simulink model "GalvoModel_v3_tfCCneu"  (R2013a)
settings: Solver=ode45  StartTime=0.0  StopTime=1.5  RelTol=1e-3
undefined symbols (not defined in the file or in its folder): BEM, ccKp, CL, CR, FR, H, KTR, RIN, TRC
libraries: simulink x1
settings Model: Creator=mainster  LastModifiedBy=mainster
settings DebuggingCC: SolverPrmCheckMsg=none

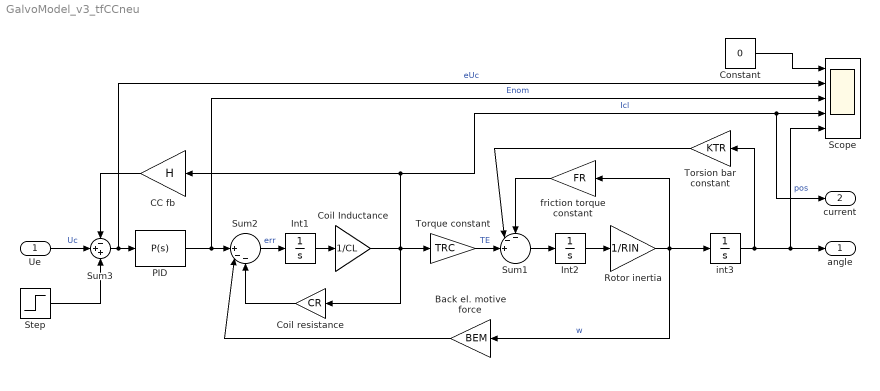
== system GalvoModel_v3_tfCCneu ==
  Ue : Inport
  Back el. motive force : Gain  Gain=BEM
  CC fb : Gain  StartFcn=|  Gain=H
      | %H=100;                       
      | sprintf('StartFcn: H is %i',H)
      settings: AttributesFormatString=H=eval(%<Gain>)
  Coil Inductance : Gain  Gain=1/CL
  Coil resistance : Gain  Gain=CR
  Constant : Constant  Value=0
  Int1 : Integrator
  Int2 : Integrator
  PID : simulink/Continuous/PID Controller  Controller=P  TimeDomain=Continuous-time  SampleTime=1  IntegratorMethod=Forward Euler  FilterMethod=Forward Euler  Form=Parallel  P=ccKp  I=1  D=0  N=100  InitialConditionSource=internal  InitialConditionForIntegrator=0  InitialConditionForFilter=0  ExternalReset=none  LimitOutput=off  UpperSaturationLimit=inf  LowerSaturationLimit=-inf  LinearizeAsGain=on  AntiWindupMode=none  Kb=1  TrackingMode=off  Kt=1  PParamMin=[]  PParamMax=[]  IParamMin=[]  IParamMax=[]  DParamMin=[]  DParamMax=[]  NParamMin=[]  NParamMax=[]  KbParamMin=[]  KbParamMax=[]  KtParamMin=[]  KtParamMax=[]  POutMin=[]  POutMax=[]  IOutMin=[]  IOutMax=[]  DOutMin=[]  DOutMax=[]  NOutMin=[]  NOutMax=[]  KbOutMin=[]  KbOutMax=[]  KtOutMin=[]  KtOutMax=[]  IntegratorOutMin=[]  IntegratorOutMax=[]  FilterOutMin=[]  FilterOutMax=[]  SumOutMin=[]  SumOutMax=[]  SumI1OutMin=[]  SumI1OutMax=[]  SumI2OutMin=[]  SumI2OutMax=[]  SumI3OutMin=[]  SumI3OutMax=[]  SumDOutMin=[]  SumDOutMax=[]  SaturationOutMin=[]  SaturationOutMax=[]  IntegratorContinuousStateAttributes=''  IntegratorStateMustResolveToSignalObject=off  IntegratorRTWStateStorageClass=Auto  FilterContinuousStateAttributes=''  FilterStateMustResolveToSignalObject=off  FilterRTWStateStorageClass=Auto
      settings: AttributesFormatString=Kp=%<P>\n%<Controller>
  Rotor inertia : Gain  Gain=1/RIN
  Scope : Scope  NumInputPorts=5
      settings: ShowLegends=on  TimeRange=1.5  YMin=-1~0.4~20~0~0  YMax=1~1~60~12~3  MaxDataPoints=500000
  Step : Step  Time=0  SampleTime=0
  Sum1 : Sum  Inputs=--+||
  Sum2 : Sum  Inputs=||+--
  Sum3 : Sum  Inputs=-++
  Torque constant : Gain  Gain=TRC
  Torsion bar constant : Gain  Gain=KTR
  friction torque constant : Gain  Gain=FR
  int3 : Integrator
  angle : Outport
  current : Outport  Port=2
  wires:
  Sum2/1 -> Int1/1  "err"
  Rotor inertia/1 -> Back el. motive force/1, int3/1, friction torque constant/1  "w"
  int3/1 -> Torsion bar constant/1, Scope/5, angle/1  "pos"
  Int1/1 -> Coil Inductance/1
  Coil resistance/1 -> Sum2/3
  Int2/1 -> Rotor inertia/1
  friction torque constant/1 -> Sum1/1
  Torsion bar constant/1 -> Sum1/2
  Torque constant/1 -> Sum1/3  "TE"
  Sum1/1 -> Int2/1
  Sum3/1 -> Scope/2, PID/1  "eUc"
  PID/1 -> Scope/3, Sum2/1  "Enom"
  Ue/1 -> Sum3/2  "Uc"
  Back el. motive force/1 -> Sum2/2
  CC fb/1 -> Sum3/1
  Step/1 -> Sum3/3
  Coil Inductance/1 -> current/1, Scope/4, CC fb/1, Coil resistance/1, Torque constant/1  "Icl"
  Constant/1 -> Scope/1
